simulink model "hdv_hydroelectropowertrain_model"  (R2026a)
settings: Solver=ode1be  StopTime=simulation_length  FixedStep=tsample  MaxStep=tsample
undefined symbols (not defined in the file): alpha, Apump, available_torque, Bpump, btheta_shaft, C1, consumption, Cpump, dp_lim, E0, E1, E2, E3, E_1, Elog, eta_v_m, eta_v_p, ki_dp_comp, ki_te_comp, kp_ctrl_m, kp_dp_comp, kp_te_comp, Kpump, load_blade_enable, Lpump, M, magnitude, Ncell, Npump, omega_e_rpm_ref, omega_l_max_rpm, q1Kalman, q2Kalman, q3Kalman, Qhr, R0, R1, R_tg, rKalman, rpm_base, rpm_consumption, simulation_length, tau_load, tau_load_max, Tc, torque_base, torque_consumption, torque_friction_base, tsample, v_track1_ref, v_track2_ref, valve_mmorifice_max, xv_m_max
libraries: fl_lib x383, nesl_utility x162, linear_swashplate_ctrl_lib x8, flexshaft_lib x5, bichamber_piston_lib x5, variable_displacement_motor_lib x4, variable_displacement_pump_lib x4, fixed_displacement_pump_lib x4, relief_valve_lib x4, inverse_shuttle_valve_lib x4, hydrostatic_threeway_valve_bichamber_piston_lib x4, hydrostatic_fourway_valve_bichamber_piston_lib x4
(part 2 of 8)

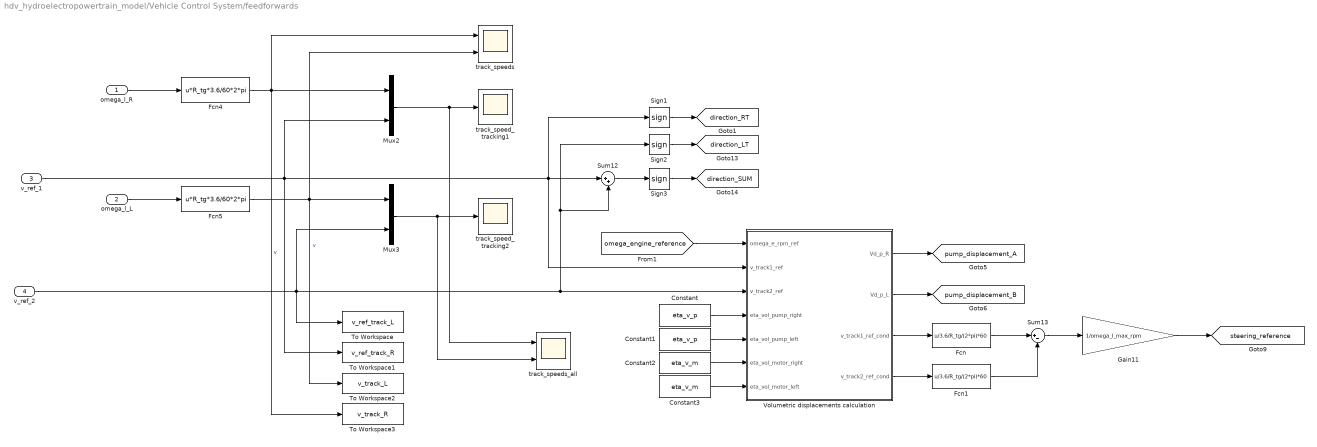
== system hdv_hydroelectropowertrain_model/Vehicle Control System/feedforwards ==
  omega_l_R : Inport
  omega_l_L : Inport  Port=2
  v_ref_1 : Inport  Port=3
  v_ref_2 : Inport  Port=4
  Constant : Constant  Value=eta_v_p
  Constant1 : Constant  Value=eta_v_p
  Constant2 : Constant  Value=eta_v_m
  Constant3 : Constant  Value=eta_v_m
  Fcn : Fcn  Expr=u/3.6/R_tg/(2*pi)*60
  Fcn1 : Fcn  Expr=u/3.6/R_tg/(2*pi)*60
  Fcn4 : Fcn  Expr=u*R_tg*3.6/60*2*pi
  Fcn5 : Fcn  Expr=u*R_tg*3.6/60*2*pi
  Gain11 : Gain  Gain=1/omega_l_max_rpm
  Mux2 : Mux  Inputs=2
  Mux3 : Mux  Inputs=2
  Sign1 : Signum
  Sign2 : Signum
  Sign3 : Signum
  Sum12 : Sum  Inputs=|++
  Sum13 : Sum  Inputs=|+-
  To Workspace : ToWorkspace  VariableName=v_ref_track_L  SampleTime=Tc
      settings: MaxDataPoints=Nc
  To Workspace1 : ToWorkspace  VariableName=v_ref_track_R  SampleTime=Tc
      settings: MaxDataPoints=Nc
  To Workspace2 : ToWorkspace  VariableName=v_track_L  SampleTime=Tc
      settings: MaxDataPoints=Nc
  To Workspace3 : ToWorkspace  VariableName=v_track_R  SampleTime=Tc
      settings: MaxDataPoints=Nc
  Volumetric displacements calculation : MATLAB Function  TreatAsAtomicUnit=on
  track_speed_tracking1 : Scope
      settings: SampleTime=tsample  ActiveDisplayYMinimum=-10.32146  ActiveDisplayYMaximum=12.89313
  track_speed_tracking2 : Scope
      settings: SampleTime=tsample  ActiveDisplayYMinimum=-13.84367  ActiveDisplayYMaximum=13.84367  DataLoggingVariableName=ScopeData2
  track_speeds : Scope  NumInputPorts=2
      settings: SampleTime=tsample  ActiveDisplayYMinimum=-9.04097  ActiveDisplayYMaximum=12.82201  DataLoggingVariableName=ScopeData3
  track_speeds_all : Scope  NumInputPorts=2
      settings: SampleTime=tsample  ActiveDisplayYMinimum=-10.03974  ActiveDisplayYMaximum=10.35769
  tag scope: direction_LT=global, direction_RT=global, direction_SUM=global, pump_displacement_A=global, pump_displacement_B=global, steering_reference=global
  wires:
  Constant3/1 -> Volumetric displacements calculation/7(eta_vol_motor_left)
  [omega_engine_reference] -> Volumetric displacements calculation/1(omega_e_rpm_ref)
  v_ref_2/1 -> To Workspace/1, Sign2/1, Sum12/2, Volumetric displacements calculation/3(v_track2_ref), Mux3/2
  v_ref_1/1 -> Mux2/2, To Workspace1/1, Volumetric displacements calculation/2(v_track1_ref), Sum12/1, Sign1/1
  Fcn/1 -> Sum13/1
  Constant/1 -> Volumetric displacements calculation/4(eta_vol_pump_right)
  Volumetric displacements calculation/4(v_track2_ref_cond) -> Fcn1/1
  Fcn5/1 -> To Workspace2/1, Mux3/1, track_speeds/2  "v"
  Constant1/1 -> Volumetric displacements calculation/5(eta_vol_pump_left)
  Sum13/1 -> Gain11/1
  Volumetric displacements calculation/3(v_track1_ref_cond) -> Fcn/1
  Sign1/1 -> [direction_RT]
  Fcn4/1 -> Mux2/1, track_speeds/1, To Workspace3/1  "v"
  Volumetric displacements calculation/1(Vd_p_R) -> [pump_displacement_A]
  Volumetric displacements calculation/2(Vd_p_L) -> [pump_displacement_B]
  omega_l_R/1 -> Fcn4/1
  Gain11/1 -> [steering_reference]
  Sign2/1 -> [direction_LT]
  Sum12/1 -> Sign3/1
  Sign3/1 -> [direction_SUM]
  Constant2/1 -> Volumetric displacements calculation/6(eta_vol_motor_right)
  Mux3/1 -> track_speeds_all/2, track_speed_tracking2/1
  Fcn1/1 -> Sum13/2
  Mux2/1 -> track_speeds_all/1, track_speed_tracking1/1
  omega_l_L/1 -> Fcn5/1

== system hdv_hydroelectropowertrain_model/Vehicle Control System/lineA_compensations ==
  Abs : Abs  SaturateOnIntegerOverflow=off
  Gain7 : Gain  Gain=-1
  Saturation Dynamic : sl_discontinuities/Saturation Dynamic  OutMin=[]  OutMax=[]  OutDataTypeStr=Inherit: Same as second input  OutDataType=fixdt(1, 16)  OutScaling=2^-10  DoSatur=off
  Sum13 : Sum  Inputs=++|
  compRT : Scope  NumInputPorts=2
      settings: SampleTime=tsample  ActiveDisplayYMinimum=-1.73756  ActiveDisplayYMaximum=1.73756  DataLoggingVariableName=ScopeData4
  direction_RT : Subsystem
  displacement_compensation : Outport
  wires:
  Saturation Dynamic/1 -> displacement_compensation/1
  Sum13/1 -> Saturation Dynamic/2
  Gain7/1 -> compRT/2, Saturation Dynamic/3
  [compensation_pressureA] -> Sum13/1
  [compensation_engine] -> direction_RT/1(In1)
  direction_RT/1(ETComp) -> Sum13/2  "engine torque compensation"
  [pump_displacement_A] -> Abs/1
  Abs/1 -> Saturation Dynamic/1, compRT/1, Gain7/1

== system hdv_hydroelectropowertrain_model/Vehicle Control System/lineB_compensations  ==
  Abs : Abs  SaturateOnIntegerOverflow=off
  Gain7 : Gain  Gain=-1
  Saturation Dynamic : sl_discontinuities/Saturation Dynamic  OutMin=[]  OutMax=[]  OutDataTypeStr=Inherit: Same as second input  OutDataType=fixdt(1, 16)  OutScaling=2^-10  DoSatur=off
  Sum12 : Sum  Inputs=|++
  compLT : Scope  NumInputPorts=2
      settings: SampleTime=tsample  ActiveDisplayYMinimum=-1.80203  ActiveDisplayYMaximum=1.80203  DataLoggingVariableName=ScopeData5
  direction_LT : Subsystem
  displacement_compensation : Outport
  wires:
  [compensation_pressureB] -> Sum12/2
  Gain7/1 -> compLT/2, Saturation Dynamic/3
  [compensation_engine] -> direction_LT/1(In1)
  direction_LT/1(ETComp) -> Sum12/1  "engine torque compensation"
  [pump_displacement_B] -> Abs/1
  Sum12/1 -> Saturation Dynamic/2
  Saturation Dynamic/1 -> displacement_compensation/1
  Abs/1 -> Saturation Dynamic/1, compLT/1, Gain7/1

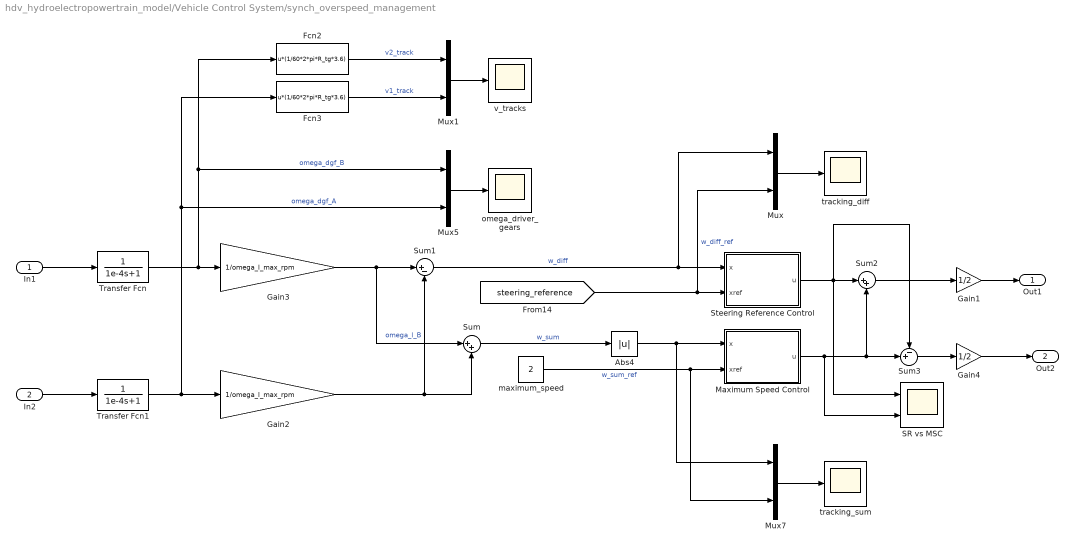
== system hdv_hydroelectropowertrain_model/Vehicle Control System/synch_overspeed_management ==
  In1 : Inport
  In2 : Inport  Port=2
  Abs4 : Abs  SaturateOnIntegerOverflow=off
  Fcn2 : Fcn  Expr=u*(1/60*2*pi*R_tg*3.6)
  Fcn3 : Fcn  Expr=u*(1/60*2*pi*R_tg*3.6)
  Gain1 : Gain  Gain=1/2
  Gain2 : Gain  Gain=1/omega_l_max_rpm
  Gain3 : Gain  Gain=1/omega_l_max_rpm
  Gain4 : Gain  Gain=1/2
  Maximum Speed Control : Subsystem  mask{kp=0.25/2, ki=4/2, ts=tsample, sat_pos=0, sat_neg=-3.28}
  Mux{,1,5,7} (4 alike) : Mux  Inputs=2
  SR vs MSC : Scope  NumInputPorts=2
      settings: SampleTime=tsample  ActiveDisplayYMinimum=-0.19705  ActiveDisplayYMaximum=0.02189  DataLoggingVariableName=ScopeData6
  Steering Reference Control : Subsystem  mask{kp=0.125 %0.5, ki=2 %8, ts=tsample, sat_pos=3.28, sat_neg=-3.28}
  Sum : Sum  Inputs=|++
  Sum1 : Sum  Inputs=|+-
  Sum2 : Sum  Inputs=|++
  Sum3 : Sum  Inputs=-+|
  Transfer Fcn : TransferFcn  Denominator=[1e-4 1]
  Transfer Fcn1 : TransferFcn  Denominator=[1e-4 1]
  maximum_speed : Constant  Value=2
  omega_driver_gears : Scope
      settings: SampleTime=tsample  ActiveDisplayYMinimum=-6.02402  ActiveDisplayYMaximum=54.18854  DataLoggingVariableName=ScopeData5
  tracking_diff : Scope
      settings: SampleTime=tsample  ActiveDisplayYMinimum=-1.6E-13  ActiveDisplayYMaximum=1.2E-13  DataLoggingVariableName=ScopeData2
  tracking_sum : Scope
      settings: SampleTime=tsample  ActiveDisplayYMinimum=-0.33251  ActiveDisplayYMaximum=2.25917
  v_tracks : Scope
      settings: SampleTime=tsample  ActiveDisplayYMinimum=-0.98977  ActiveDisplayYMaximum=8.90333
  Out1 : Outport
  Out2 : Outport  Port=2
  wires:
  Mux7/1 -> tracking_sum/1
  Sum/1 -> Abs4/1  "w_sum"
  Gain3/1 -> Sum/1, Sum1/1
  Mux1/1 -> v_tracks/1
  maximum_speed/1 -> Maximum Speed Control/2(xref), Mux7/2  "w_sum_ref"
  Sum3/1 -> Gain4/1
  Sum1/1 -> Mux/1, Steering Reference Control/1(x)  "w_diff"
  Transfer Fcn/1 -> Fcn2/1, Mux5/1, Gain3/1  "omega_dgf_B"
  Maximum Speed Control/1(u) -> SR vs MSC/2, Sum2/2, Sum3/2
  Gain2/1 -> Sum1/2, Sum/2  "omega_l_B"
  In1/1 -> Transfer Fcn/1
  Mux/1 -> tracking_diff/1
  Gain1/1 -> Out1/1
  Sum2/1 -> Gain1/1
  Mux5/1 -> omega_driver_gears/1
  Abs4/1 -> Mux7/1, Maximum Speed Control/1(x)
  Fcn3/1 -> Mux1/2  "v1_track"
  [steering_reference] -> Mux/2, Steering Reference Control/2(xref)  "w_diff_ref"
  Steering Reference Control/1(u) -> Sum3/1, SR vs MSC/1, Sum2/1
  Transfer Fcn1/1 -> Fcn3/1, Mux5/2, Gain2/1  "omega_dgf_A"
  Fcn2/1 -> Mux1/1  "v2_track"
  Gain4/1 -> Out2/1
  In2/1 -> Transfer Fcn1/1

== system hdv_hydroelectropowertrain_model/Vehicle Control System/tracks references ==
  Manual Switch : ManualSwitch
  Manual Switch1 : ManualSwitch  CurrentSetting=0
  Repeating Sequence Stair1 : simulink/Sources/Repeating Sequence Stair  OutValues=[v_track2_ref -v_track2_ref v_track2_ref -v_track2_ref v_track2_ref -v_track2_ref].'  tsamp=floor(simulation_length/6)  OutMin=[]  OutMax=[]  OutDataTypeStr=double  OutputDataTypeScalingMode=double  OutDataType=fixdt(0,8)  ConRadixGroup=Best Precision: Vector-wise  OutScaling=2^-12
  Repeating Sequence Stair2 : simulink/Sources/Repeating Sequence Stair  OutValues=[v_track1_ref -v_track1_ref v_track1_ref -v_track1_ref v_track1_ref -v_track1_ref].'  tsamp=floor(simulation_length/6)  OutMin=[]  OutMax=[]  OutDataTypeStr=double  OutputDataTypeScalingMode=double  OutDataType=fixdt(0,8)  ConRadixGroup=Best Precision: Vector-wise  OutScaling=2^-12
  Sum : Sum  Inputs=|++
  Sum1 : Sum  Inputs=++|
  v_track1_ref : Step  Time=10  FinalValue=v_track1_ref  SampleTime=0
  v_track1_ref1 : Step  Time=simulation_length/2  FinalValue=-2*v_track1_ref  SampleTime=0
  v_track2_ref : Step  Time=10  FinalValue=v_track2_ref  SampleTime=0
  v_track2_ref1 : Step  Time=simulation_length/2  FinalValue=-2*v_track2_ref  SampleTime=0
  speed_track_1_ref : Outport
  speed_track_2_ref : Outport  Port=2
  wires:
  v_track1_ref1/1 -> Sum1/1
  v_track2_ref1/1 -> Sum/2
  v_track1_ref/1 -> Sum1/2
  v_track2_ref/1 -> Sum/1
  Manual Switch/1 -> speed_track_1_ref/1
  Manual Switch1/1 -> speed_track_2_ref/1
  Sum1/1 -> Manual Switch/2
  Sum/1 -> Manual Switch1/1
  Repeating Sequence Stair2/1 -> Manual Switch/1
  Repeating Sequence Stair1/1 -> Manual Switch1/2

== system hdv_hydroelectropowertrain_model/external_load/loadA ==
  Rate Limiter : RateLimiter  RisingSlewLimit=tau_load_max/5  FallingSlewLimit=-tau_load_max/5  SampleTimeMode=inherited
  Saturation : Saturate  UpperLimit=abs(tau_load)  LowerLimit=-abs(tau_load)
  Step : Step  Time=5  FinalValue=tau_load  SampleTime=0
  Out1 : Outport
  wires:
  Saturation/1 -> Out1/1
  Rate Limiter/1 -> Saturation/1
  Step/1 -> Rate Limiter/1

== system hdv_hydroelectropowertrain_model/external_load/loadB ==
  Rate Limiter : RateLimiter  RisingSlewLimit=tau_load_max/5  FallingSlewLimit=-tau_load_max/5  SampleTimeMode=inherited
  Saturation : Saturate  UpperLimit=abs(tau_load)  LowerLimit=-abs(tau_load)
  Step : Step  Time=5  FinalValue=tau_load  SampleTime=0
  Out1 : Outport
  wires:
  Step/1 -> Rate Limiter/1
  Rate Limiter/1 -> Saturation/1
  Saturation/1 -> Out1/1

== system hdv_hydroelectropowertrain_model/PR776_powertrain/Hydrostatic_powertrain/driveine_LD1 ==
  Connection Label1 : ConnectionLabel  Label=pS1
  Connection Label2 : ConnectionLabel  Label=pS1
  Connection Label3 : ConnectionLabel  Label=pT1
  Connection Label4 : ConnectionLabel  Label=pS2
  Connection Label5 : ConnectionLabel  Label=pT2
  Connection Label6 : ConnectionLabel  Label=pT1
  Connection Label7 : ConnectionLabel  Label=pS2
  Connection Label8 : ConnectionLabel  Label=pT2
  Variable displacement motor LD : variable_displacement_motor_lib/Variable displacement motor  max_Dv=Vm_nom cm^3/rev  min_Dv=20 cm^3/rev  inertia_motor=0.0402 kg*m^2  oil_vol=4.1 l  bp=b1 N*m/(rad/s)  lk=1e-6 m  t_specify=off  t_priority=None  t=0 N*m  t_nominal_specify=off  t_nominal_value=1  t_nominal_unit=N*m  q_specify=off  q_priority=None  q=0 m^3/s  q_nominal_specify=off  q_nominal_value=1  q_nominal_unit=m^3/s  qt_specify=off  qt_priority=None  qt=0 m^3/s  qt_nominal_specify=off  qt_nominal_value=1  qt_nominal_unit=m^3/s  qleak_specify=off  qleak_priority=None  qleak=0 m^3/s  qleak_nominal_specify=off  qleak_nominal_value=1  qleak_nominal_unit=m^3/s  Dv_specify=off  Dv_priority=None  Dv=0 cm^3/rev  Dv_nominal_specify=off  Dv_nominal_value=1  Dv_nominal_unit=cm^3/rev  dp_specify=off  dp_priority=None  dp=0 Pa  dp_nominal_specify=off  dp_nominal_value=1  dp_nominal_unit=Pa  wm_specify=off  wm_priority=None  wm=0 rad/s  wm_nominal_specify=off  wm_nominal_value=1  wm_nominal_unit=rad/s
  Variable displacement pump LD : variable_displacement_pump_lib/Variable displacement pump  max_Dv=Vp_nom cm^3/rev  inertia_pump=0.027 kg*m^2  oil_vol=3.0 l  bp=b1 N*m/(rad/s)  lk=1e-6 m  t_specify=off  t_priority=None  t=0 N*m  t_nominal_specify=off  t_nominal_value=1  t_nominal_unit=N*m  q_specify=off  q_priority=None  q=0 m^3/s  q_nominal_specify=off  q_nominal_value=1  q_nominal_unit=m^3/s  qt_specify=off  qt_priority=None  qt=0 m^3/s  qt_nominal_specify=off  qt_nominal_value=1  qt_nominal_unit=m^3/s  qleak_specify=off  qleak_priority=None  qleak=0 m^3/s  qleak_nominal_specify=off  qleak_nominal_value=1  qleak_nominal_unit=m^3/s  Dv_specify=off  Dv_priority=None  Dv=0 cm^3/rev  Dv_nominal_specify=off  Dv_nominal_value=1  Dv_nominal_unit=cm^3/rev  dp_specify=off  dp_priority=None  dp=0 Pa  dp_nominal_specify=off  dp_nominal_value=1  dp_nominal_unit=Pa  we_specify=off  we_priority=None  we=0 rad/s  we_nominal_specify=off  we_nominal_value=1  we_nominal_unit=rad/s
  flexible shaft1 : flexshaft_lib/flexible shaft  b1=b1 N*m/(rad/s)  J1=J1 kg*m^2  b2=b2 N*m/(rad/s)  J2=J2 kg*m^2  b_theta=b_theta N*m/(rad/s)  k_theta=k_theta N*m/rad  w_1_specify=off  w_1_priority=None  w_1=0 rad/s  w_1_nominal_specify=off  w_1_nominal_value=1  w_1_nominal_unit=rad/s  w_2_specify=off  w_2_priority=None  w_2=0 rad/s  w_2_nominal_specify=off  w_2_nominal_value=1  w_2_nominal_unit=rad/s  t_1_specify=off  t_1_priority=None  t_1=0 N*m  t_1_nominal_specify=off  t_1_nominal_value=1  t_1_nominal_unit=N*m  t_2_specify=off  t_2_priority=None  t_2=0 N*m  t_2_nominal_specify=off  t_2_nominal_value=1  t_2_nominal_unit=N*m  t_theta_specify=off  t_theta_priority=None  t_theta=0 N*m  t_theta_nominal_specify=off  t_theta_nominal_value=1  t_theta_nominal_unit=N*m
  pressure_charge_system_LD : Subsystem
      settings: PortSchema="{\"entries\":[{\"content\":{\"sides\":[{\"content\":{\"connectorIds\":[]},\"type\":\"ConnectorPlacement.EquallySpacedRectSide\",\"uuid\":\"e48dc60c-7abd-410a-894b-273047c8aadd\"},{\"content\":{\"connectorIds\":[],\"side\":\"RIGHT\"},\"type\":\"ConnectorPlacement.EquallySpacedRectSide\",\"uuid\":\"1866d745-b28e-4187-be81-03bff766c239\"},{\"content\":{\"connectorIds\":[\"LConn1\"],\"side\":\"TOP\"},\"type\":\"ConnectorPlacement.EquallySpacedRectSide\",\"uuid\":\"a7856f22-1a7f-4c46-a37a-59c4b01a6b79\"},{\"content\":{\"connectorIds\":[\"RConn1\",\"RConn2\"],\"side\":\"BOTTOM\"},\"type\":\"ConnectorPlacement.EquallySpacedRectSide\",\"uuid\":\"6254cc6e-0892-4919-86d5-0180151530d1\"}]},\"type\":\"ConnectorPlacement.EquallySpacedConnector\",\"uuid\":\"a983534e-afc0-4bb2-9b1c-06b03353b26b\"}],\"packageUris\":[\"http://schema.mathworks.com/mf0/Connector/19700101\"],\"version\":\"1.0\"}"
  vd_ctrl_motor_LD : Subsystem
  vd_ctrl_pump_LD : Subsystem
  s : PMIOPort  Side=Left
  pS1 : PMIOPort  Port=2  Side=Left
  pS2 : PMIOPort  Port=3  Side=Left
  pT1 : PMIOPort  Port=4  Side=Left
  pT2 : PMIOPort  Port=5  Side=Left
  q : PMIOPort  Port=6  Side=Right
  dp : PMIOPort  Port=7  Side=Right
  c : PMIOPort  Port=8  Side=Right
  RDA : PMIOPort  Port=9  Side=Right
  RDB : PMIOPort  Port=10  Side=Right
  wires:
  [DpB] -> vd_ctrl_pump_LD/1(vd_ref)
  [DmB] -> vd_ctrl_motor_LD/1(vd_ref)
  connections:
  flexible shaft1/LConn1 -- s/RConn1
  Variable displacement pump LD/RConn1 -- RDA/RConn1 -- Variable displacement motor LD/LConn2 -- pressure_charge_system_LD/LConn1
  vd_ctrl_pump_LD/RConn1 -- Variable displacement pump LD/LConn1
  vd_ctrl_pump_LD/LConn1 -- Connection Label2/LConn1
  flexible shaft1/RConn1 -- pressure_charge_system_LD/RConn2 -- Variable displacement pump LD/LConn2
  vd_ctrl_motor_LD/RConn1 -- Variable displacement motor LD/LConn1
  vd_ctrl_pump_LD/LConn2 -- Connection Label3/LConn1
  Connection Label4/LConn1 -- vd_ctrl_motor_LD/LConn1
  Connection Label5/LConn1 -- vd_ctrl_motor_LD/LConn2
  Variable displacement motor LD/LConn3 -- pressure_charge_system_LD/RConn1 -- Variable displacement pump LD/RConn2 -- RDB/RConn1
  Variable displacement motor LD/RConn2 -- q/RConn1
  Variable displacement motor LD/RConn3 -- dp/RConn1
  c/RConn1 -- Variable displacement motor LD/RConn1
  pS2/RConn1 -- Connection Label7/LConn1
  pS1/RConn1 -- Connection Label1/LConn1
  pT1/RConn1 -- Connection Label6/LConn1
  pT2/RConn1 -- Connection Label8/LConn1

== system hdv_hydroelectropowertrain_model/PR776_powertrain/Hydrostatic_powertrain/driveine_LD2 ==
  Connection Label1 : ConnectionLabel  Label=pS1
  Connection Label2 : ConnectionLabel  Label=pS1
  Connection Label3 : ConnectionLabel  Label=pT1
  Connection Label4 : ConnectionLabel  Label=pS2
  Connection Label5 : ConnectionLabel  Label=pT2
  Connection Label6 : ConnectionLabel  Label=pT1
  Connection Label7 : ConnectionLabel  Label=pS2
  Connection Label8 : ConnectionLabel  Label=pT2
  Variable displacement motor LD : variable_displacement_motor_lib/Variable displacement motor  max_Dv=Vm_nom cm^3/rev  min_Dv=20 cm^3/rev  inertia_motor=0.0402 kg*m^2  oil_vol=4.1 l  bp=b1 N*m/(rad/s)  lk=1e-6 m  t_specify=off  t_priority=None  t=0 N*m  t_nominal_specify=off  t_nominal_value=1  t_nominal_unit=N*m  q_specify=off  q_priority=None  q=0 m^3/s  q_nominal_specify=off  q_nominal_value=1  q_nominal_unit=m^3/s  qt_specify=off  qt_priority=None  qt=0 m^3/s  qt_nominal_specify=off  qt_nominal_value=1  qt_nominal_unit=m^3/s  qleak_specify=off  qleak_priority=None  qleak=0 m^3/s  qleak_nominal_specify=off  qleak_nominal_value=1  qleak_nominal_unit=m^3/s  Dv_specify=off  Dv_priority=None  Dv=0 cm^3/rev  Dv_nominal_specify=off  Dv_nominal_value=1  Dv_nominal_unit=cm^3/rev  dp_specify=off  dp_priority=None  dp=0 Pa  dp_nominal_specify=off  dp_nominal_value=1  dp_nominal_unit=Pa  wm_specify=off  wm_priority=None  wm=0 rad/s  wm_nominal_specify=off  wm_nominal_value=1  wm_nominal_unit=rad/s
  Variable displacement pump LD : variable_displacement_pump_lib/Variable displacement pump  max_Dv=Vp_nom cm^3/rev  inertia_pump=0.027 kg*m^2  oil_vol=3.0 l  bp=b1 N*m/(rad/s)  lk=1e-6 m  t_specify=off  t_priority=None  t=0 N*m  t_nominal_specify=off  t_nominal_value=1  t_nominal_unit=N*m  q_specify=off  q_priority=None  q=0 m^3/s  q_nominal_specify=off  q_nominal_value=1  q_nominal_unit=m^3/s  qt_specify=off  qt_priority=None  qt=0 m^3/s  qt_nominal_specify=off  qt_nominal_value=1  qt_nominal_unit=m^3/s  qleak_specify=off  qleak_priority=None  qleak=0 m^3/s  qleak_nominal_specify=off  qleak_nominal_value=1  qleak_nominal_unit=m^3/s  Dv_specify=off  Dv_priority=None  Dv=0 cm^3/rev  Dv_nominal_specify=off  Dv_nominal_value=1  Dv_nominal_unit=cm^3/rev  dp_specify=off  dp_priority=None  dp=0 Pa  dp_nominal_specify=off  dp_nominal_value=1  dp_nominal_unit=Pa  we_specify=off  we_priority=None  we=0 rad/s  we_nominal_specify=off  we_nominal_value=1  we_nominal_unit=rad/s
  flexible shaft1 : flexshaft_lib/flexible shaft  b1=b1 N*m/(rad/s)  J1=J1 kg*m^2  b2=b2 N*m/(rad/s)  J2=J2 kg*m^2  b_theta=b_theta N*m/(rad/s)  k_theta=k_theta N*m/rad  w_1_specify=off  w_1_priority=None  w_1=0 rad/s  w_1_nominal_specify=off  w_1_nominal_value=1  w_1_nominal_unit=rad/s  w_2_specify=off  w_2_priority=None  w_2=0 rad/s  w_2_nominal_specify=off  w_2_nominal_value=1  w_2_nominal_unit=rad/s  t_1_specify=off  t_1_priority=None  t_1=0 N*m  t_1_nominal_specify=off  t_1_nominal_value=1  t_1_nominal_unit=N*m  t_2_specify=off  t_2_priority=None  t_2=0 N*m  t_2_nominal_specify=off  t_2_nominal_value=1  t_2_nominal_unit=N*m  t_theta_specify=off  t_theta_priority=None  t_theta=0 N*m  t_theta_nominal_specify=off  t_theta_nominal_value=1  t_theta_nominal_unit=N*m
  pressure_charge_system_LD : Subsystem
      settings: PortSchema="{\"entries\":[{\"content\":{\"sides\":[{\"content\":{\"connectorIds\":[]},\"type\":\"ConnectorPlacement.EquallySpacedRectSide\",\"uuid\":\"e48dc60c-7abd-410a-894b-273047c8aadd\"},{\"content\":{\"connectorIds\":[],\"side\":\"RIGHT\"},\"type\":\"ConnectorPlacement.EquallySpacedRectSide\",\"uuid\":\"1866d745-b28e-4187-be81-03bff766c239\"},{\"content\":{\"connectorIds\":[\"LConn1\"],\"side\":\"TOP\"},\"type\":\"ConnectorPlacement.EquallySpacedRectSide\",\"uuid\":\"a7856f22-1a7f-4c46-a37a-59c4b01a6b79\"},{\"content\":{\"connectorIds\":[\"RConn1\",\"RConn2\"],\"side\":\"BOTTOM\"},\"type\":\"ConnectorPlacement.EquallySpacedRectSide\",\"uuid\":\"6254cc6e-0892-4919-86d5-0180151530d1\"}]},\"type\":\"ConnectorPlacement.EquallySpacedConnector\",\"uuid\":\"a983534e-afc0-4bb2-9b1c-06b03353b26b\"}],\"packageUris\":[\"http://schema.mathworks.com/mf0/Connector/19700101\"],\"version\":\"1.0\"}"
  vd_ctrl_motor_LD : Subsystem
  vd_ctrl_pump_LD : Subsystem
  s : PMIOPort  Side=Left
  pS1 : PMIOPort  Port=2  Side=Left
  pS2 : PMIOPort  Port=3  Side=Left
  pT1 : PMIOPort  Port=4  Side=Left
  pT2 : PMIOPort  Port=5  Side=Left
  q : PMIOPort  Port=6  Side=Right
  dp : PMIOPort  Port=7  Side=Right
  c : PMIOPort  Port=8  Side=Right
  RDA : PMIOPort  Port=9  Side=Right
  RDB : PMIOPort  Port=10  Side=Right
  wires:
  [DmB] -> vd_ctrl_motor_LD/1(vd_ref)
  [DpB] -> vd_ctrl_pump_LD/1(vd_ref)
  connections:
  pT2/RConn1 -- Connection Label8/LConn1
  pT1/RConn1 -- Connection Label6/LConn1
  pS1/RConn1 -- Connection Label1/LConn1
  pS2/RConn1 -- Connection Label7/LConn1
  c/RConn1 -- Variable displacement motor LD/RConn1
  Variable displacement motor LD/RConn3 -- dp/RConn1
  Variable displacement motor LD/RConn2 -- q/RConn1
  pressure_charge_system_LD/RConn1 -- Variable displacement motor LD/LConn3 -- RDB/RConn1 -- Variable displacement pump LD/RConn2
  Connection Label5/LConn1 -- vd_ctrl_motor_LD/LConn2
  Connection Label4/LConn1 -- vd_ctrl_motor_LD/LConn1
  vd_ctrl_pump_LD/LConn2 -- Connection Label3/LConn1
  vd_ctrl_motor_LD/RConn1 -- Variable displacement motor LD/LConn1
  Variable displacement pump LD/LConn2 -- pressure_charge_system_LD/RConn2 -- flexible shaft1/RConn1
  vd_ctrl_pump_LD/LConn1 -- Connection Label2/LConn1
  vd_ctrl_pump_LD/RConn1 -- Variable displacement pump LD/LConn1
  pressure_charge_system_LD/LConn1 -- RDA/RConn1 -- Variable displacement pump LD/RConn1 -- Variable displacement motor LD/LConn2
  flexible shaft1/LConn1 -- s/RConn1

== system hdv_hydroelectropowertrain_model/PR776_powertrain/Hydrostatic_powertrain/driveine_RD1 ==
  Connection Label1 : ConnectionLabel  Label=pS1
  Connection Label2 : ConnectionLabel  Label=pT1
  Connection Label3 : ConnectionLabel  Label=pS2
  Connection Label4 : ConnectionLabel  Label=pT2
  Connection Label6 : ConnectionLabel  Label=pS1
  Connection Label7 : ConnectionLabel  Label=pT1
  Connection Label8 : ConnectionLabel  Label=pS2
  Connection Label9 : ConnectionLabel  Label=pT2
  Variable displacement motor RD : variable_displacement_motor_lib/Variable displacement motor  max_Dv=Vm_nom cm^3/rev  min_Dv=20 cm^3/rev  inertia_motor=0.0402 kg*m^2  oil_vol=4.1 l  bp=b1 N*m/(rad/s)  lk=1e-6 m  t_specify=off  t_priority=None  t=0 N*m  t_nominal_specify=off  t_nominal_value=1  t_nominal_unit=N*m  q_specify=off  q_priority=None  q=0 m^3/s  q_nominal_specify=off  q_nominal_value=1  q_nominal_unit=m^3/s  qt_specify=off  qt_priority=None  qt=0 m^3/s  qt_nominal_specify=off  qt_nominal_value=1  qt_nominal_unit=m^3/s  qleak_specify=off  qleak_priority=None  qleak=0 m^3/s  qleak_nominal_specify=off  qleak_nominal_value=1  qleak_nominal_unit=m^3/s  Dv_specify=off  Dv_priority=None  Dv=0 cm^3/rev  Dv_nominal_specify=off  Dv_nominal_value=1  Dv_nominal_unit=cm^3/rev  dp_specify=off  dp_priority=None  dp=0 Pa  dp_nominal_specify=off  dp_nominal_value=1  dp_nominal_unit=Pa  wm_specify=off  wm_priority=None  wm=0 rad/s  wm_nominal_specify=off  wm_nominal_value=1  wm_nominal_unit=rad/s
  Variable displacement pump RD : variable_displacement_pump_lib/Variable displacement pump  max_Dv=Vp_nom cm^3/rev  inertia_pump=0.027 kg*m^2  oil_vol=3.0 l  bp=b1 N*m/(rad/s)  lk=1e-6 m  t_specify=off  t_priority=None  t=0 N*m  t_nominal_specify=off  t_nominal_value=1  t_nominal_unit=N*m  q_specify=off  q_priority=None  q=0 m^3/s  q_nominal_specify=off  q_nominal_value=1  q_nominal_unit=m^3/s  qt_specify=off  qt_priority=None  qt=0 m^3/s  qt_nominal_specify=off  qt_nominal_value=1  qt_nominal_unit=m^3/s  qleak_specify=off  qleak_priority=None  qleak=0 m^3/s  qleak_nominal_specify=off  qleak_nominal_value=1  qleak_nominal_unit=m^3/s  Dv_specify=off  Dv_priority=None  Dv=0 cm^3/rev  Dv_nominal_specify=off  Dv_nominal_value=1  Dv_nominal_unit=cm^3/rev  dp_specify=off  dp_priority=None  dp=0 Pa  dp_nominal_specify=off  dp_nominal_value=1  dp_nominal_unit=Pa  we_specify=off  we_priority=None  we=0 rad/s  we_nominal_specify=off  we_nominal_value=1  we_nominal_unit=rad/s
  flexible shaft2 : flexshaft_lib/flexible shaft  b1=b1 N*m/(rad/s)  J1=J1 kg*m^2  b2=b2 N*m/(rad/s)  J2=J2 kg*m^2  b_theta=b_theta N*m/(rad/s)  k_theta=k_theta N*m/rad  w_1_specify=off  w_1_priority=None  w_1=0 rad/s  w_1_nominal_specify=off  w_1_nominal_value=1  w_1_nominal_unit=rad/s  w_2_specify=off  w_2_priority=None  w_2=0 rad/s  w_2_nominal_specify=off  w_2_nominal_value=1  w_2_nominal_unit=rad/s  t_1_specify=off  t_1_priority=None  t_1=0 N*m  t_1_nominal_specify=off  t_1_nominal_value=1  t_1_nominal_unit=N*m  t_2_specify=off  t_2_priority=None  t_2=0 N*m  t_2_nominal_specify=off  t_2_nominal_value=1  t_2_nominal_unit=N*m  t_theta_specify=off  t_theta_priority=None  t_theta=0 N*m  t_theta_nominal_specify=off  t_theta_nominal_value=1  t_theta_nominal_unit=N*m
  pressure_charge_system_RD : Subsystem
      settings: PortSchema="{\"entries\":[{\"content\":{\"sides\":[{\"content\":{\"connectorIds\":[]},\"type\":\"ConnectorPlacement.EquallySpacedRectSide\",\"uuid\":\"e48dc60c-7abd-410a-894b-273047c8aadd\"},{\"content\":{\"connectorIds\":[],\"side\":\"RIGHT\"},\"type\":\"ConnectorPlacement.EquallySpacedRectSide\",\"uuid\":\"1866d745-b28e-4187-be81-03bff766c239\"},{\"content\":{\"connectorIds\":[\"LConn1\"],\"side\":\"TOP\"},\"type\":\"ConnectorPlacement.EquallySpacedRectSide\",\"uuid\":\"a7856f22-1a7f-4c46-a37a-59c4b01a6b79\"},{\"content\":{\"connectorIds\":[\"RConn1\",\"RConn2\"],\"side\":\"BOTTOM\"},\"type\":\"ConnectorPlacement.EquallySpacedRectSide\",\"uuid\":\"6254cc6e-0892-4919-86d5-0180151530d1\"}]},\"type\":\"ConnectorPlacement.EquallySpacedConnector\",\"uuid\":\"a983534e-afc0-4bb2-9b1c-06b03353b26b\"}],\"packageUris\":[\"http://schema.mathworks.com/mf0/Connector/19700101\"],\"version\":\"1.0\"}"
  vd_ctrl_motor_RD : Subsystem
  vd_ctrl_pump_RD : Subsystem
  s : PMIOPort  Side=Left
  q : PMIOPort  Port=2  Side=Right
  dp : PMIOPort  Port=3  Side=Right
  c : PMIOPort  Port=4  Side=Right
  pS1 : PMIOPort  Port=5  Side=Left
  pS2 : PMIOPort  Port=6  Side=Left
  pT1 : PMIOPort  Port=7  Side=Left
  pT2 : PMIOPort  Port=8  Side=Left
  RDA : PMIOPort  Port=9  Side=Right
  RDB : PMIOPort  Port=10  Side=Right
  wires:
  [DmA] -> vd_ctrl_motor_RD/1(vd_ref)
  [DpA] -> vd_ctrl_pump_RD/1(vd_ref)
  connections:
  Variable displacement motor RD/LConn3 -- pressure_charge_system_RD/RConn1 -- RDB/RConn1 -- Variable displacement pump RD/RConn2
  Connection Label7/LConn1 -- vd_ctrl_pump_RD/LConn2
  flexible shaft2/RConn1 -- pressure_charge_system_RD/RConn2 -- Variable displacement pump RD/LConn2
  Connection Label6/LConn1 -- vd_ctrl_pump_RD/LConn1
  vd_ctrl_motor_RD/RConn1 -- Variable displacement motor RD/LConn1
  vd_ctrl_motor_RD/LConn2 -- Connection Label9/LConn1
  vd_ctrl_motor_RD/LConn1 -- Connection Label8/LConn1
  Variable displacement pump RD/RConn1 -- RDA/RConn1 -- Variable displacement motor RD/LConn2 -- pressure_charge_system_RD/LConn1
  vd_ctrl_pump_RD/RConn1 -- Variable displacement pump RD/LConn1
  s/RConn1 -- flexible shaft2/LConn1
  Variable displacement motor RD/RConn2 -- q/RConn1
  Variable displacement motor RD/RConn1 -- c/RConn1
  Variable displacement motor RD/RConn3 -- dp/RConn1
  pS1/RConn1 -- Connection Label1/LConn1
  pT1/RConn1 -- Connection Label2/LConn1
  pS2/RConn1 -- Connection Label3/LConn1
  pT2/RConn1 -- Connection Label4/LConn1

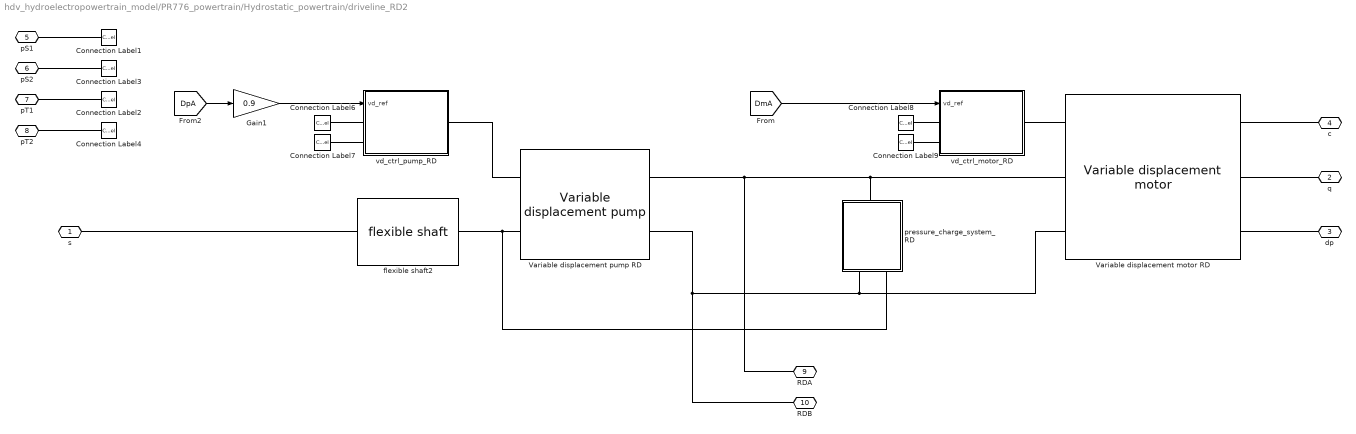
== system hdv_hydroelectropowertrain_model/PR776_powertrain/Hydrostatic_powertrain/driveline_RD2 ==
  Connection Label1 : ConnectionLabel  Label=pS1
  Connection Label2 : ConnectionLabel  Label=pT1
  Connection Label3 : ConnectionLabel  Label=pS2
  Connection Label4 : ConnectionLabel  Label=pT2
  Connection Label6 : ConnectionLabel  Label=pS1
  Connection Label7 : ConnectionLabel  Label=pT1
  Connection Label8 : ConnectionLabel  Label=pS2
  Connection Label9 : ConnectionLabel  Label=pT2
  Gain1 : Gain  Gain=0.9
  Variable displacement motor RD : variable_displacement_motor_lib/Variable displacement motor  max_Dv=Vm_nom cm^3/rev  min_Dv=20 cm^3/rev  inertia_motor=0.0402 kg*m^2  oil_vol=4.1 l  bp=b1 N*m/(rad/s)  lk=1e-6 m  t_specify=off  t_priority=None  t=0 N*m  t_nominal_specify=off  t_nominal_value=1  t_nominal_unit=N*m  q_specify=off  q_priority=None  q=0 m^3/s  q_nominal_specify=off  q_nominal_value=1  q_nominal_unit=m^3/s  qt_specify=off  qt_priority=None  qt=0 m^3/s  qt_nominal_specify=off  qt_nominal_value=1  qt_nominal_unit=m^3/s  qleak_specify=off  qleak_priority=None  qleak=0 m^3/s  qleak_nominal_specify=off  qleak_nominal_value=1  qleak_nominal_unit=m^3/s  Dv_specify=off  Dv_priority=None  Dv=0 cm^3/rev  Dv_nominal_specify=off  Dv_nominal_value=1  Dv_nominal_unit=cm^3/rev  dp_specify=off  dp_priority=None  dp=0 Pa  dp_nominal_specify=off  dp_nominal_value=1  dp_nominal_unit=Pa  wm_specify=off  wm_priority=None  wm=0 rad/s  wm_nominal_specify=off  wm_nominal_value=1  wm_nominal_unit=rad/s
  Variable displacement pump RD : variable_displacement_pump_lib/Variable displacement pump  max_Dv=Vp_nom cm^3/rev  inertia_pump=0.027 kg*m^2  oil_vol=3.0 l  bp=b1 N*m/(rad/s)  lk=1e-6 m  t_specify=off  t_priority=None  t=0 N*m  t_nominal_specify=off  t_nominal_value=1  t_nominal_unit=N*m  q_specify=off  q_priority=None  q=0 m^3/s  q_nominal_specify=off  q_nominal_value=1  q_nominal_unit=m^3/s  qt_specify=off  qt_priority=None  qt=0 m^3/s  qt_nominal_specify=off  qt_nominal_value=1  qt_nominal_unit=m^3/s  qleak_specify=off  qleak_priority=None  qleak=0 m^3/s  qleak_nominal_specify=off  qleak_nominal_value=1  qleak_nominal_unit=m^3/s  Dv_specify=off  Dv_priority=None  Dv=0 cm^3/rev  Dv_nominal_specify=off  Dv_nominal_value=1  Dv_nominal_unit=cm^3/rev  dp_specify=off  dp_priority=None  dp=0 Pa  dp_nominal_specify=off  dp_nominal_value=1  dp_nominal_unit=Pa  we_specify=off  we_priority=None  we=0 rad/s  we_nominal_specify=off  we_nominal_value=1  we_nominal_unit=rad/s
  flexible shaft2 : flexshaft_lib/flexible shaft  b1=b1 N*m/(rad/s)  J1=J1 kg*m^2  b2=b2 N*m/(rad/s)  J2=J2 kg*m^2  b_theta=b_theta N*m/(rad/s)  k_theta=k_theta N*m/rad  w_1_specify=off  w_1_priority=None  w_1=0 rad/s  w_1_nominal_specify=off  w_1_nominal_value=1  w_1_nominal_unit=rad/s  w_2_specify=off  w_2_priority=None  w_2=0 rad/s  w_2_nominal_specify=off  w_2_nominal_value=1  w_2_nominal_unit=rad/s  t_1_specify=off  t_1_priority=None  t_1=0 N*m  t_1_nominal_specify=off  t_1_nominal_value=1  t_1_nominal_unit=N*m  t_2_specify=off  t_2_priority=None  t_2=0 N*m  t_2_nominal_specify=off  t_2_nominal_value=1  t_2_nominal_unit=N*m  t_theta_specify=off  t_theta_priority=None  t_theta=0 N*m  t_theta_nominal_specify=off  t_theta_nominal_value=1  t_theta_nominal_unit=N*m
  pressure_charge_system_RD : Subsystem
      settings: PortSchema="{\"entries\":[{\"content\":{\"sides\":[{\"content\":{\"connectorIds\":[]},\"type\":\"ConnectorPlacement.EquallySpacedRectSide\",\"uuid\":\"e48dc60c-7abd-410a-894b-273047c8aadd\"},{\"content\":{\"connectorIds\":[],\"side\":\"RIGHT\"},\"type\":\"ConnectorPlacement.EquallySpacedRectSide\",\"uuid\":\"1866d745-b28e-4187-be81-03bff766c239\"},{\"content\":{\"connectorIds\":[\"LConn1\"],\"side\":\"TOP\"},\"type\":\"ConnectorPlacement.EquallySpacedRectSide\",\"uuid\":\"a7856f22-1a7f-4c46-a37a-59c4b01a6b79\"},{\"content\":{\"connectorIds\":[\"RConn1\",\"RConn2\"],\"side\":\"BOTTOM\"},\"type\":\"ConnectorPlacement.EquallySpacedRectSide\",\"uuid\":\"6254cc6e-0892-4919-86d5-0180151530d1\"}]},\"type\":\"ConnectorPlacement.EquallySpacedConnector\",\"uuid\":\"a983534e-afc0-4bb2-9b1c-06b03353b26b\"}],\"packageUris\":[\"http://schema.mathworks.com/mf0/Connector/19700101\"],\"version\":\"1.0\"}"
  vd_ctrl_motor_RD : Subsystem
  vd_ctrl_pump_RD : Subsystem
  s : PMIOPort  Side=Left
  q : PMIOPort  Port=2  Side=Right
  dp : PMIOPort  Port=3  Side=Right
  c : PMIOPort  Port=4  Side=Right
  pS1 : PMIOPort  Port=5  Side=Left
  pS2 : PMIOPort  Port=6  Side=Left
  pT1 : PMIOPort  Port=7  Side=Left
  pT2 : PMIOPort  Port=8  Side=Left
  RDA : PMIOPort  Port=9  Side=Right
  RDB : PMIOPort  Port=10  Side=Right
  wires:
  [DmA] -> vd_ctrl_motor_RD/1(vd_ref)
  [DpA] -> Gain1/1
  Gain1/1 -> vd_ctrl_pump_RD/1(vd_ref)
  connections:
  pT2/RConn1 -- Connection Label4/LConn1
  pS2/RConn1 -- Connection Label3/LConn1
  pT1/RConn1 -- Connection Label2/LConn1
  pS1/RConn1 -- Connection Label1/LConn1
  Variable displacement motor RD/RConn3 -- dp/RConn1
  Variable displacement motor RD/RConn1 -- c/RConn1
  Variable displacement motor RD/RConn2 -- q/RConn1
  s/RConn1 -- flexible shaft2/LConn1
  vd_ctrl_pump_RD/RConn1 -- Variable displacement pump RD/LConn1
  pressure_charge_system_RD/LConn1 -- RDA/RConn1 -- Variable displacement pump RD/RConn1 -- Variable displacement motor RD/LConn2
  vd_ctrl_motor_RD/LConn1 -- Connection Label8/LConn1
  vd_ctrl_motor_RD/LConn2 -- Connection Label9/LConn1
  vd_ctrl_motor_RD/RConn1 -- Variable displacement motor RD/LConn1
  Connection Label6/LConn1 -- vd_ctrl_pump_RD/LConn1
  Variable displacement pump RD/LConn2 -- pressure_charge_system_RD/RConn2 -- flexible shaft2/RConn1
  Connection Label7/LConn1 -- vd_ctrl_pump_RD/LConn2
  pressure_charge_system_RD/RConn1 -- Variable displacement motor RD/LConn3 -- RDB/RConn1 -- Variable displacement pump RD/RConn2

== system hdv_hydroelectropowertrain_model/PR776_powertrain/constant_pressure_source/Pressure controlled pump ==
  Hydraulic Flow Rate Sensor : fl_lib/Hydraulic/Hydraulic Sensors/Hydraulic Flow Rate Sensor
  Hydraulic Pressure Sensor : fl_lib/Hydraulic/Hydraulic Sensors/Hydraulic Pressure Sensor
  Hydraulic Reference : fl_lib/Hydraulic/Hydraulic Elements/Hydraulic Reference
  PS Step : fl_lib/Physical Signals/Sources/PS Step  step_time=20 s  initial_value=32 bar  final_value=32 bar
  PS-Simulink Converter : nesl_utility/PS-Simulink Converter  PhysicalDomain=network_engine_domain  SubClassName=ps_output  LeftPortType=input  RightPortType=output  PseudoPeriodic=off  Frequencies=[]  VectorFormat=1-D array  Unit=bar  AffineConversion=on
  PS-Simulink Converter1 : nesl_utility/PS-Simulink Converter  PhysicalDomain=network_engine_domain  SubClassName=ps_output  LeftPortType=input  RightPortType=output  PseudoPeriodic=off  Frequencies=[]  VectorFormat=1-D array  Unit=l/min  AffineConversion=on
  PS-Simulink Converter{2..5} (4 alike) : nesl_utility/PS-Simulink Converter  PhysicalDomain=network_engine_domain  SubClassName=ps_output  LeftPortType=input  RightPortType=output  PseudoPeriodic=off  Frequencies=[]  VectorFormat=1-D array  Unit=1  AffineConversion=off
  Pressure controlled pump : pressure_controlled_pump_lib/Pressure controlled pump  Vd_nom=62.3 cm^3/rev  pnom=32 bar  b=0.1 N*m/(rad/s)  inertia_pump=0.027 kg*m^2  vd_lim_max=0.98  vd_lim_min=0  p_set=258 bar  p_reg=8 bar  x_rv_max=12 mm  kpc=2  kic=40 1/s  te_specify=off  te_priority=None  te=0 N*m  te_nominal_specify=off  te_nominal_value=1  te_nominal_unit=N*m  qA_specify=off  qA_priority=None  qA=0 m^3/s  qA_nominal_specify=off  qA_nominal_value=1  qA_nominal_unit=m^3/s  qB_specify=off  qB_priority=None  qB=0 m^3/s  qB_nominal_specify=off  qB_nominal_value=1  qB_nominal_unit=m^3/s  qd_specify=off  qd_priority=None  qd=0 m^3/s  qd_nominal_specify=off  qd_nominal_value=1  qd_nominal_unit=m^3/s  dp_specify=off  dp_priority=None  dp=0 Pa  dp_nominal_specify=off  dp_nominal_value=1  dp_nominal_unit=Pa  vd_specify=off  vd_priority=None  vd=0  vd_nominal_specify=off  vd_nominal_value=1  vd_nominal_unit=1  vd_i_specify=off  vd_i_priority=None  vd_i=0  vd_i_nominal_specify=off  vd_i_nominal_value=1  vd_i_nominal_unit=1  we_specify=off  we_priority=None  we=0 rad/s  we_nominal_specify=off  we_nominal_value=1  we_nominal_unit=rad/s
  flow : Scope
      settings: ActiveDisplayYMinimum=-14.44491  ActiveDisplayYMaximum=32.0327
  leak/ptorque : Scope  NumInputPorts=3
      settings: ActiveDisplayYMinimum=-0.13628  ActiveDisplayYMaximum=1.22651  DataLoggingVariableName=ScopeData2
  pressure : Scope
      settings: ActiveDisplayYMinimum=-4.33344  ActiveDisplayYMaximum=39.00093
  pump_flow : Scope
      settings: ActiveDisplayYMinimum=-110.85023  ActiveDisplayYMaximum=12.31659  DataLoggingVariableName=ScopeData4
  pS : PMIOPort  Side=Right
  shaft : PMIOPort  Port=2  Side=Left
  pT : PMIOPort  Port=3  Side=Right
  wires:
  PS-Simulink Converter/1 -> pressure/1
  PS-Simulink Converter2/1 -> leak/ptorque/1  "leak"
  PS-Simulink Converter5/1 -> pump_flow/1
  PS-Simulink Converter3/1 -> leak/ptorque/2  "torque"
  PS-Simulink Converter4/1 -> leak/ptorque/3  "vd"
  PS-Simulink Converter1/1 -> flow/1
  connections:
  PS-Simulink Converter/LConn1 -- Hydraulic Pressure Sensor/RConn2
  Pressure controlled pump/RConn6 -- PS-Simulink Converter5/LConn1
  Pressure controlled pump/RConn5 -- PS-Simulink Converter4/LConn1
  Pressure controlled pump/RConn1 -- Hydraulic Flow Rate Sensor/LConn1
  Hydraulic Pressure Sensor/RConn1 -- pT/RConn1 -- Pressure controlled pump/RConn2 -- Hydraulic Reference/LConn1
  Hydraulic Flow Rate Sensor/RConn2 -- pS/RConn1 -- Hydraulic Pressure Sensor/LConn1
  Hydraulic Flow Rate Sensor/RConn1 -- PS-Simulink Converter1/LConn1
  Pressure controlled pump/RConn3 -- PS-Simulink Converter2/LConn1
  Pressure controlled pump/RConn4 -- PS-Simulink Converter3/LConn1
  shaft/RConn1 -- Pressure controlled pump/LConn1
  PS Step/RConn1 -- Pressure controlled pump/LConn2

== system hdv_hydroelectropowertrain_model/PR776_powertrain/constant_pressure_source/Pressure controlled pump1 ==
  Hydraulic Flow Rate Sensor : fl_lib/Hydraulic/Hydraulic Sensors/Hydraulic Flow Rate Sensor
  Hydraulic Pressure Sensor : fl_lib/Hydraulic/Hydraulic Sensors/Hydraulic Pressure Sensor
  Hydraulic Reference : fl_lib/Hydraulic/Hydraulic Elements/Hydraulic Reference
  PS Constant : fl_lib/Physical Signals/Sources/PS Constant  constant=250 bar
  PS-Simulink Converter : nesl_utility/PS-Simulink Converter  PhysicalDomain=network_engine_domain  SubClassName=ps_output  LeftPortType=input  RightPortType=output  PseudoPeriodic=off  Frequencies=[]  VectorFormat=1-D array  Unit=bar  AffineConversion=on
  PS-Simulink Converter1 : nesl_utility/PS-Simulink Converter  PhysicalDomain=network_engine_domain  SubClassName=ps_output  LeftPortType=input  RightPortType=output  PseudoPeriodic=off  Frequencies=[]  VectorFormat=1-D array  Unit=l/min  AffineConversion=on
  PS-Simulink Converter{2..5} (4 alike) : nesl_utility/PS-Simulink Converter  PhysicalDomain=network_engine_domain  SubClassName=ps_output  LeftPortType=input  RightPortType=output  PseudoPeriodic=off  Frequencies=[]  VectorFormat=1-D array  Unit=1  AffineConversion=off
  Pressure controlled pump : pressure_controlled_pump_lib/Pressure controlled pump  Vd_nom=62.3*4 cm^3/rev  pnom=250 bar  b=0.1 N*m/(rad/s)  inertia_pump=0.027 kg*m^2  vd_lim_max=0.98  vd_lim_min=0  p_set=258 bar  p_reg=8 bar  x_rv_max=12 mm  kpc=2  kic=40 1/s  te_specify=off  te_priority=None  te=0 N*m  te_nominal_specify=off  te_nominal_value=1  te_nominal_unit=N*m  qA_specify=off  qA_priority=None  qA=0 m^3/s  qA_nominal_specify=off  qA_nominal_value=1  qA_nominal_unit=m^3/s  qB_specify=off  qB_priority=None  qB=0 m^3/s  qB_nominal_specify=off  qB_nominal_value=1  qB_nominal_unit=m^3/s  qd_specify=off  qd_priority=None  qd=0 m^3/s  qd_nominal_specify=off  qd_nominal_value=1  qd_nominal_unit=m^3/s  dp_specify=off  dp_priority=None  dp=0 Pa  dp_nominal_specify=off  dp_nominal_value=1  dp_nominal_unit=Pa  vd_specify=off  vd_priority=None  vd=0  vd_nominal_specify=off  vd_nominal_value=1  vd_nominal_unit=1  vd_i_specify=off  vd_i_priority=None  vd_i=0  vd_i_nominal_specify=off  vd_i_nominal_value=1  vd_i_nominal_unit=1  we_specify=off  we_priority=None  we=0 rad/s  we_nominal_specify=off  we_nominal_value=1  we_nominal_unit=rad/s
  flow : Scope
      settings: ActiveDisplayYMinimum=-14.44491  ActiveDisplayYMaximum=32.0327
  leak/ptorque : Scope  NumInputPorts=3
      settings: ActiveDisplayYMinimum=-0.00579  ActiveDisplayYMaximum=0.0038  DataLoggingVariableName=ScopeData2
  pressure : Scope
      settings: ActiveDisplayYMinimum=230.17764  ActiveDisplayYMaximum=276.69408
  pump_flow : Scope
      settings: ActiveDisplayYMinimum=-110.85023  ActiveDisplayYMaximum=12.31659  DataLoggingVariableName=ScopeData4
  pS : PMIOPort  Side=Right
  shaft : PMIOPort  Port=2  Side=Left
  pT : PMIOPort  Port=3  Side=Right
  wires:
  PS-Simulink Converter1/1 -> flow/1
  PS-Simulink Converter4/1 -> leak/ptorque/3  "vd"
  PS-Simulink Converter3/1 -> leak/ptorque/2  "torque"
  PS-Simulink Converter5/1 -> pump_flow/1
  PS-Simulink Converter2/1 -> leak/ptorque/1  "leak"
  PS-Simulink Converter/1 -> pressure/1
  connections:
  shaft/RConn1 -- Pressure controlled pump/LConn1
  Pressure controlled pump/RConn4 -- PS-Simulink Converter3/LConn1
  Pressure controlled pump/RConn3 -- PS-Simulink Converter2/LConn1
  Hydraulic Flow Rate Sensor/RConn1 -- PS-Simulink Converter1/LConn1
  Hydraulic Pressure Sensor/LConn1 -- pS/RConn1 -- Hydraulic Flow Rate Sensor/RConn2
  Hydraulic Reference/LConn1 -- Pressure controlled pump/RConn2 -- pT/RConn1 -- Hydraulic Pressure Sensor/RConn1
  Pressure controlled pump/RConn1 -- Hydraulic Flow Rate Sensor/LConn1
  Pressure controlled pump/RConn5 -- PS-Simulink Converter4/LConn1
  Pressure controlled pump/RConn6 -- PS-Simulink Converter5/LConn1
  PS-Simulink Converter/LConn1 -- Hydraulic Pressure Sensor/RConn2
  PS Constant/RConn1 -- Pressure controlled pump/LConn2

== system hdv_hydroelectropowertrain_model/PR776_powertrain/electrical_main_drive_train/LithiumIonBattery ==
  Bus Creator : BusCreator  Inputs=4
  Current Sensor : fl_lib/Electrical/Electrical Sensors/Current Sensor
  Current Sensor1 : fl_lib/Electrical/Electrical Sensors/Current Sensor
  Electrical Reference1 : fl_lib/Electrical/Electrical Elements/Electrical Reference
  PS-Simulink Converter1 : nesl_utility/PS-Simulink Converter  PhysicalDomain=network_engine_domain  SubClassName=ps_output  LeftPortType=input  RightPortType=output  PseudoPeriodic=off  Frequencies=[]  VectorFormat=1-D array  Unit=1  AffineConversion=off
  PS-Simulink Converter4 : nesl_utility/PS-Simulink Converter  PhysicalDomain=network_engine_domain  SubClassName=ps_output  LeftPortType=input  RightPortType=output  PseudoPeriodic=off  Frequencies=[]  VectorFormat=1-D array  Unit=1  AffineConversion=off
  PS-Simulink Converter5 : nesl_utility/PS-Simulink Converter  PhysicalDomain=network_engine_domain  SubClassName=ps_output  LeftPortType=input  RightPortType=output  PseudoPeriodic=off  Frequencies=[]  VectorFormat=1-D array  Unit=V  AffineConversion=on
  Resistor1 : fl_lib/Electrical/Electrical Elements/Resistor  R=1e4 Ohm  i_specify=off  i_priority=None  i=0 A  i_nominal_specify=off  i_nominal_value=1  i_nominal_unit=A  v_specify=off  v_priority=None  v=0 V  v_nominal_specify=off  v_nominal_value=1  v_nominal_unit=V
  Resistor2 : fl_lib/Electrical/Electrical Elements/Resistor  R=1e4 Ohm  i_specify=off  i_priority=None  i=0 A  i_nominal_specify=off  i_nominal_value=1  i_nominal_unit=A  v_specify=off  v_priority=None  v=0 V  v_nominal_specify=off  v_nominal_value=1  v_nominal_unit=V
  Unit Delay5 : UnitDelay  SampleTime=tsample
  Voltage Sensor : fl_lib/Electrical/Electrical Sensors/Voltage Sensor
  lithium ion cell analytical ocv : Subsystem
  Uout+ : PMIOPort  Side=Right
  Uout- : PMIOPort  Port=2  Side=Right
  Uin+ : PMIOPort  Port=3  Side=Left
  Uin- : PMIOPort  Port=4  Side=Left
  lithiumIonBattery_Data : Outport
  tag scope: vout_battery=global
  wires:
  PS-Simulink Converter5/1 -> Unit Delay5/1
  PS-Simulink Converter4/1 -> [iout_battery]  "i batt"
  Unit Delay5/1 -> [vout_battery]
  Bus Creator/1 -> lithiumIonBattery_Data/1
  [iout_battery] -> Bus Creator/1  "Iout_battery"
  [vout_battery] -> Bus Creator/2  "Vout_battery"
  [soc_battery] -> Bus Creator/3  "soc_battery"
  PS-Simulink Converter1/1 -> [iin_battery]  "i batt"
  [iin_battery] -> Bus Creator/4  "iin_battery"
  connections:
  Current Sensor/RConn1 -- PS-Simulink Converter4/LConn1
  Current Sensor/RConn2 -- Voltage Sensor/LConn1 -- Resistor2/LConn1 -- Uout+/RConn1
  Voltage Sensor/RConn1 -- PS-Simulink Converter5/LConn1
  Voltage Sensor/RConn2 -- Resistor1/RConn1 -- Uin-/RConn1 -- Electrical Reference1/LConn1 -- lithium ion cell analytical ocv/RConn2 -- Resistor2/RConn1 -- Uout-/RConn1
  lithium ion cell analytical ocv/RConn1 -- Current Sensor1/RConn2 -- Current Sensor/LConn1
  Current Sensor1/RConn1 -- PS-Simulink Converter1/LConn1
  Uin+/RConn1 -- Resistor1/LConn1 -- Current Sensor1/LConn1
